simulink model "ModeAdjust"  (R2018b)
settings: Solver=FixedStepDiscrete  StartTime=0.0  StopTime=inf  FixedStep=0.01  RelTol=1e-3
undefined symbols (not defined in the file or in its folder): IfKeSMSbSeatMovBkRclnEnable_Val, IfKeSMSbSeatMovFrwdBkwdEnable_Val, IfKeSMSbSeatMovFtrstEnable_Val, IfKeSMSbSeatMovHdrstFrwdBkwdEnable_Val, IfKeSMSbSeatMovHdUpwdDnwdEnable_Val, IfKeSMSbSeatMovLgrstEnable_Val, IfKeSMSbSeatMovLtwdRtwdEnable_Val, IfVeSMSeStNumConfig, KeSMSbArmscreenMovEnable_Val, KeSMSbSeatMovLgrstExpdEnable_Val, KeSMSuFirstRwStBackPosDelta_Val, KeSMSuFirstRwStBackPosTolr_Val, KeSMSuFirstRwStCushFrntPosDelta_Val, KeSMSuFirstRwStCushFrntPosTolr_Val, KeSMSuFirstRwStCushRePosDelta_Val, KeSMSuFirstRwStCushRePosTolr_Val, KeSMSuFirstRwStFootrestPosDelta_Val, KeSMSuFirstRwStFootrestPosTolr_Val, KeSMSuFirstRwStFwdBkwdPosDelta_Val, KeSMSuFirstRwStFwdBkwdPosTolr_Val, KeSMSuMdMotFinshdTm_Val, KeSMSuMdRetryTm1_Val, KeSMSuModeReqDurgTm_Val, KeSMSuSecRwStArmTochPosDelta_Val, KeSMSuSecRwStArmTochPosTolr_Val, KeSMSuSecRwStBackPosDelta_Val, KeSMSuSecRwStBackPosTolr_Val, KeSMSuSecRwStFtrstUpwdDnwdPosDelta_Val, KeSMSuSecRwStFtrstUpwdDnwdPosTolr_Val, KeSMSuSecRwStFwdBkwdPosDelta_Val, KeSMSuSecRwStFwdBkwdPosTolr_Val, KeSMSuSecRwStHeadrestFwdBkwdPosDelta_Val, KeSMSuSecRwStHeadrestFwdBkwdPosTolr_Val, KeSMSuSecRwStHeadrestUpwdDwnwdPosDelta_Val, KeSMSuSecRwStHeadrestUpwdDwnwdPosTolr_Val, KeSMSuSecRwStLegrestInOutPosDelta_Val, KeSMSuSecRwStLegrestInOutPosTolr_Val, KeSMSuSecRwStLegrestUpwdDwnwdPosDelta_Val, KeSMSuSecRwStLegrestUpwdDwnwdPosTolr_Val, KeSMSuSecRwStLwdRwdPosDelta_Val, KeSMSuSecRwStLwdRwdPosTolr_Val, KeSMSuSecRwStVIPFtrstRefAngle_Val, KeSMSuThirdRwStFwdBkwdPosDelta_Val, KeSMSuThirdRwStFwdBkwdPosTolr_Val, KeSMSuThrdRwCushFoldPosDelta_Val, KeSMSuThrdRwCushFoldPosTolr_Val, KeSMSuThrdRwStBackPosDelta_Val, KeSMSuThrdRwStBackPosTolr_Val, KeSMSw4SLegrstCloseMdSecRwLtStFtrstUpwdDnwdPos_Val, KeSMSw4SLegrstCloseMdSecRwLtStFtrstUpwdDnwdPosMax_Val, KeSMSw4SLegrstCloseMdSecRwLtStFtrstUpwdDnwdPosMin_Val, KeSMSw4SLegrstCloseMdSecRwLtStLgrstOtwdInwdPos_Val, KeSMSw4SLegrstCloseMdSecRwLtStLgrstOtwdInwdPosMax_Val, KeSMSw4SLegrstCloseMdSecRwLtStLgrstOtwdInwdPosMin_Val, KeSMSw4SLegrstCloseMdSecRwLtStLgrstUpwdDnwdPos_Val, KeSMSw4SLegrstCloseMdSecRwLtStLgrstUpwdDnwdPosMax_Val, KeSMSw4SLegrstCloseMdSecRwLtStLgrstUpwdDnwdPosMin_Val, KeSMSw4SLegrstCloseMdSecRwRtStFtrstUpwdDnwdPos_Val, KeSMSw4SLegrstCloseMdSecRwRtStFtrstUpwdDnwdPosMax_Val, KeSMSw4SLegrstCloseMdSecRwRtStFtrstUpwdDnwdPosMin_Val ... (+1138)
libraries: Lib x401
(part 4 of 35)

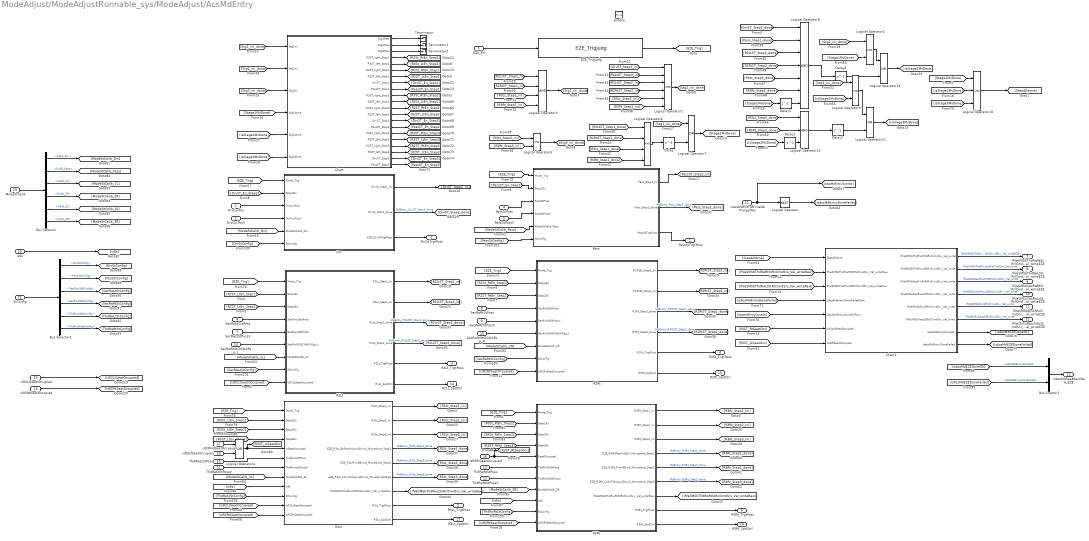
== system ModeAdjust/ModeAdjustRunnable_sys/ModeAdjust/AcsMdEntry ==
  EZE_En : Inport
  DrvCurPos : Inport  Port=2
  DrvCurPosV : Inport  Port=3
  PassStPoss : Inport  Port=4
  PassStPossV : Inport  Port=5
  SecRwLtStsPoss : Inport  Port=6
  SecRwLtStPossV : Inport  Port=7
  SecRwRtStPoss : Inport  Port=8
  SecRwRtStPossV : Inport  Port=9
  ThdRwLtStPoss : Inport  Port=10
  ThdRwLtStPossV : Inport  Port=11
  ThdRwRtStPoss : Inport  Port=12
  ThdRwRtStPossV : Inport  Port=13
  SecRwRtStChldLkRsp_L : Inport  Port=14
  SecRwRtStChldLkRsp_R : Inport  Port=15
  isR3RtSeatOccupied : Inport  Port=16
  isR3MidSeatOccupied : Inport  Port=17
  isR3LfSeatOccupied : Inport  Port=18
  ModeStCalib : Inport  Port=19
  is6s : Inport  Port=20
  StConfig : Inport  Port=21
  isAcsMdEntryArrivedAtTargetPos : Inport  Port=22
  isR2LtSeatOccupied : Inport  Port=23
  isR2RtSeatOccupied : Inport  Port=24
  Enable : EnablePort  StatesWhenEnabling=reset
  Bus Creator1 : BusCreator  Inputs=2
  Bus Selector : BusSelector  OutputSignals=Calib_Drv,Calib_Pass,Calib_2L,Calib_2R,Calib_3L,Calib_3R
  Bus Selector1 : BusSelector  OutputSignals=DrvStConfig,PassStConfig,SecRwLtStConfig,SecRwRtStConfig,ThdRwLtStConfig,ThdRwRtStConfig
  Chart : Stateflow chart  TreatAsAtomicUnit=on
  Chart1 : Stateflow chart  TreatAsAtomicUnit=on
  Delay{,1..4} (5 alike) : Delay  DelayLength=1
  Drv : Subsystem
  EZE_TrigJudg : Lib/EZE_TrigJudg  SystemSampleTime=-1
  Logical Operator : Logic  Operator=NOT  AllPortsSameDT=off  OutDataTypeStr=boolean
  Logical Operator1 : Logic  AllPortsSameDT=off  OutDataTypeStr=boolean
  Logical Operator{4,7,11,13} (4 alike) : Logic  Operator=OR  AllPortsSameDT=off  OutDataTypeStr=boolean
  Logical Operator12 : Logic  Inputs=3  AllPortsSameDT=off  OutDataTypeStr=boolean
  Logical Operator16 : Logic  Inputs=3  AllPortsSameDT=off  OutDataTypeStr=boolean
  Logical Operator2 : Logic  Inputs=6  AllPortsSameDT=off  OutDataTypeStr=boolean
  Logical Operator3 : Logic  Inputs=4  AllPortsSameDT=off  OutDataTypeStr=boolean
  Logical Operator5 : Logic  AllPortsSameDT=off  OutDataTypeStr=boolean
  Logical Operator6 : Logic  Inputs=4  AllPortsSameDT=off  OutDataTypeStr=boolean
  Logical Operator8 : Logic  Inputs=7  AllPortsSameDT=off  OutDataTypeStr=boolean
  Logical Operator9 : Logic  AllPortsSameDT=off  OutDataTypeStr=boolean
  Pass : Subsystem
  R2Lt : Subsystem
  R2Rt : Subsystem
  R3Lt : Subsystem
  R3Rt : Subsystem
  Terminator : Terminator
  Terminator1 : Terminator
  Terminator2 : Terminator
  DrvStTrgtPoss : Outport  VectorParamsAs1DForOutWhenUnconnected=on
  PassStTrgtPoss : Outport  Port=2  VectorParamsAs1DForOutWhenUnconnected=on
  R2Lt_TrgtPoss : Outport  Port=3  VectorParamsAs1DForOutWhenUnconnected=on
  R2Rt_TrgtPoss : Outport  Port=4  VectorParamsAs1DForOutWhenUnconnected=on
  R3Lt_TrgtPoss : Outport  Port=5  VectorParamsAs1DForOutWhenUnconnected=on
  R3Rt_TrgtPoss : Outport  Port=6  VectorParamsAs1DForOutWhenUnconnected=on
  IfVeSMSbThdRwRtStRclCmdSrv_Val_writeEZE : Outport  Port=7
  IfVeSMSbThdRwLtStRclCmdSrv_Val_writeEZE : Outport  Port=8
  IfVeSMSbSecRwRtStRclCmdSrv_Val_writeEZE : Outport  Port=9
  IfVeSMSuSecRwLtStRclCmdSrv_Val_writeEZE : Outport  Port=10
  IfVeSMSbDrvStRclCmdSrv_Val_writeEZE : Outport  Port=11
  IfVeSMSuPassStRclCmdSrv_Val_writeEZE : Outport  Port=12
  isAcsMdFeedBackNew_EZE : Outport  Port=13
  R2Lt_SpdCtrl : Outport  Port=14
  R2Rt_SpdCtrl : Outport  Port=15
  R3Rt_SpdCtrl : Outport  Port=16
  R3Lt_SpdCtrl : Outport  Port=17
  wires:
  EZE_En/1 -> EZE_TrigJudg/1
  EZE_TrigJudg/1 -> [EZE_Trig]
  [EZE_Trig] -> R3Rt/1(Mode_Trig)
  isR3LfSeatOccupied/1 -> Logical Operator4/2
  Logical Operator4/1 -> [R3ST_LtSeatOcc], R3Lt/5(isSeatOccupied)
  R3Rt/1(R3Rt_Step1_ini) -> [R3Rt_Step1_ini]
  R3Lt/1(R3Lt_Step1_ini) -> [R3Lt_Step1_ini]
  [Stg2_ini_done] -> Chart/2(Stg2ini)
  Chart/4(R3ST_right_Step1) -> [R3St_RtEn_Step1]
  [Stg1_ini_done] -> Chart/1(Stg1ini)
  [isStage3MvDone] -> Chart/6(Stg3done)
  [isStage2MvDone] -> Chart/5(Stg2done)
  [Stg3_ini_done] -> Chart/3(Stg3ini)
  [Stage1MvDone] -> Chart/4(Stg1done)
  Logical Operator5/1 -> [Stg3_ini_done]
  Logical Operator2/1 -> [Stg2_ini_done]
  Logical Operator3/1 -> [Stg1_ini_done]
  Chart/7(R2ST_left_Step1) -> [R2ST_LtEn_Step1]
  Chart/5(R3ST_left_Step1) -> [R3St_LtEn_Step1]
  Chart/6(R2ST_right_Step1) -> [R2St_RtEn_Step1]
  Chart/8(DrvST_Step1) -> [DrvST_En_Step1]
  Chart/9(PassST_Step1) -> [PassST_En_Step1]
  [PassST_En_Step2] -> Pass/2(Step1En)
  Logical Operator11/1 -> [isStage3MvDone]
  Logical Operator6/1 -> Delay/1
  Logical Operator7/1 -> [Stage1MvDone]
  [Stg1_ini_done] -> Logical Operator7/1
  Logical Operator13/1 -> [isStage2MvDone]
  Delay/1 -> Logical Operator7/2
  Logical Operator12/1 -> Delay2/1
  [R3Lt_Step3_done] -> Logical Operator12/1
  [R3Rt_Step3_done] -> Logical Operator12/2
  Logical Operator8/1 -> Delay4/1
  Drv/1(DrvSt_Step1_ini) -> [DrvST_Step2_ini]
  Pass/1(Pass_Step1_ini) -> [PassST_Step2_ini]
  R2Lt/1(R2Lt_Step1_Ini) -> [R2LtST_Step1_ini]
  R2Rt/1(R2RtSt_Step1_ini) -> [R2RtST_Step1_ini]
  R2Lt/2(R2Lt_Step2_Ini) -> [R2LtST_Step2_ini]
  R2Rt/2(R2RtSt_Step2_ini) -> [R2RtST_Step2_ini]
  R3Lt/2(R3Lt_Step2_ini) -> [R3Lt_Step2_ini]
  R3Rt/2(R3Rt_Step2_ini) -> [R3Rt_Step2_ini]
  R3Lt/3(R3Lt_Step3_ini) -> [R3Lt_Step3_ini]
  R3Rt/3(R3Rt_Step3_ini) -> [R3Rt_Step3_ini]
  [R3Lt_Step3_ini] -> Logical Operator5/1
  [R3Rt_Step3_ini] -> Logical Operator5/2
  Drv/2(DrvSt_Step1_done) -> [DrvST_Step2_done]  "MdEntry_DrvST_Step1_done"
  Pass/2(Pass_Step1_done) -> [Pass_Step2_done]  "MdEntry_Pass_Step1_done"
  R2Lt/3(R2Lt_Step1_done) -> [R2LtST_Step1_done]  "MdEntry_R2LtST_Step1_done"
  R2Lt/4(R2Lt_Step2_done) -> [R2LtST_Step2_done]  "MdEntry_R2LtST_Step2_done"
  R2Rt/3(R2Rt_Step1_done) -> [R2RtST_Step1_done]  "MdEntry_R2RtST_Step1_done"
  R2Rt/4(R2Rt_Step2_done) -> [R2RtST_Step2_done]  "MdEntry_R2RtST_Step2_done"
  R3Lt/4(EZE_R3Lt_BkReclnUpwdDnwd_Movedone_Step1) -> [R3Lt_Step1_done]  "MdEntry_R3Lt_Step1_done"
  R3Lt/5(EZE_R3LtFrwdBkwd_Movedone_Step2) -> [R3Lt_Step2_done]  "MdEntry_R3Lt_Step2_done"
  R3Lt/6(EZE_R3Lt_CshnFldUpwdDnwd_MovedoneStep3) -> [R3Lt_Step3_done]  "MdEntry_R3Lt_Step3_done"
  R3Rt/4(EZE_R3RtReclnUpDn_Movedone_Step1) -> [R3Rt_Step1_done]  "MdEntry_R3Rt_Step1_done"
  R3Rt/5(EZE_R3Rt_FrwdBkwd_Movedone_Step2) -> [R3Rt_Step2_done]  "MdEntry_R3Rt_Step2_done"
  R3Rt/6(EZE_R3Rt_CshnFldUpwdDnwd_Movedone_Step3) -> [R3Rt_Step3_done]  "MdEntry_R3Rt_Step3_done"
  [R2LtST_Step2_done] -> Logical Operator8/3
  [R3Lt_Step2_done] -> Logical Operator8/5
  [R3Rt_Step2_done] -> Logical Operator8/6
  R3Rt/7(IfVeSMSbThdRwRtStRclCmdSrv_Val_writeRaw) -> [IfVeSMSbThdRwRtStRclCmdSrv_Val_writeRaw]
  [IfVeSMSbThdRwRtStRclCmdSrv_Val_writeRaw] -> Chart1/2(IfVeSMSbThdRwRtStRclCmdSrv_Val_writeRaw)
  R3Lt/7(IfVeSMSbThdRwLtStRclCmdSrv_Val_writeRaw) -> [IfVeSMSbThdRwLtStRclCmdSrv_Val_writeRaw]
  [IfVeSMSbThdRwLtStRclCmdSrv_Val_writeRaw] -> Chart1/3(IfVeSMSbThdRwLtStRclCmdSrv_Val_writeRaw)
  [StepAlldone] -> Chart1/1(StepAlldone)
  Chart1/1(IfVeSMSbThdRwRtStRclCmdSrv_Val_write) -> IfVeSMSbThdRwRtStRclCmdSrv_Val_writeEZE/1  "IfVeSMSbThdRwRtStRclCmdSrv_Val_writeEZE"
  Chart1/2(IfVeSMSbThdRwLtStRclCmdSrv_Val_write) -> IfVeSMSbThdRwLtStRclCmdSrv_Val_writeEZE/1  "IfVeSMSbThdRwLtStRclCmdSrv_Val_write"
  Chart1/3(IfVeSMSbSecRwRtStRclCmdSrv_Val_write) -> IfVeSMSbSecRwRtStRclCmdSrv_Val_writeEZE/1  "IfVeSMSbSecRwRtStRclCmdSrv_Val_write"
  Chart1/4(IfVeSMSuSecRwLtStRclCmdSrv_Val_write) -> IfVeSMSuSecRwLtStRclCmdSrv_Val_writeEZE/1  "IfVeSMSuSecRwLtStRclCmdSrv_Val_write"
  Chart1/5(IfVeSMSbDrvStRclCmdSrv_Val_write) -> IfVeSMSbDrvStRclCmdSrv_Val_writeEZE/1  "IfVeSMSbDrvStRclCmdSrv_Val_write"
  Chart1/6(IfVeSMSuPassStRclCmdSrv_Val_write) -> IfVeSMSuPassStRclCmdSrv_Val_writeEZE/1  "IfVeSMSuPassStRclCmdSrv_Val_write"
  Chart/1(Stg1Req) -> Terminator/1
  Chart/2(Stg2Req) -> Terminator1/1
  Chart/3(Stg3Req) -> Terminator2/1
  isAcsMdEntryArrivedAtTargetPos/1 -> [isAcsMdEntryDoneOk], Logical Operator/1
  [isAcsMdEntryDoneOk] -> Chart1/5(isAcsMdEntryDoneOkRaw)
  [isAcsMdEntryDoneFailed] -> Chart1/4(isAcsMdEntryDoneFailedRaw)
  Chart1/7(isAcsMdEntryDoneOk) -> [isAcsMdEZEDoneOk]
  [EZE_Trig] -> Drv/1(Mode_Trig)
  [EZE_Trig] -> Pass/1(Mode_Trig)
  [EZE_Trig] -> R2Rt/1(Mode_Trig)
  [EZE_Trig] -> R2Lt/1(Mode_Trig)
  Drv/3(EZE_DrvStTrgtPoss) -> DrvStTrgtPoss/1
  Pass/3(PassStTrgtPoss) -> PassStTrgtPoss/1
  R2Lt/5(R2Lt_TrgtPoss) -> R2Lt_TrgtPoss/1
  R2Rt/5(R2Rt_TrgtPoss) -> R2Rt_TrgtPoss/1
  R3Lt/8(R3Lt_TrgtPoss) -> R3Lt_TrgtPoss/1
  [EZE_Trig] -> R3Lt/1(Mode_Trig)
  R3Rt/8(R3Rt_TrgtPoss) -> R3Rt_TrgtPoss/1
  DrvCurPos/1 -> Drv/3(DrvCurPos)
  DrvCurPosV/1 -> Drv/4(DrvCurPosV)
  PassStPoss/1 -> Pass/3(PassStPoss)
  PassStPossV/1 -> Pass/4(PassStPossV)
  SecRwLtStsPoss/1 -> R2Lt/4(SecRwLtStsPoss)
  SecRwLtStPossV/1 -> R2Lt/5(SecRwLtStPossV)
  ThdRwLtStPoss/1 -> R3Lt/6(ThdRwLtStPoss)
  ThdRwLtStPossV/1 -> R3Lt/7(ThdRwLtStPossV)
  ThdRwRtStPoss/1 -> R3Rt/6(ThdRwRtStPoss)
  ThdRwRtStPossV/1 -> R3Rt/7(ThdRwRtStPossV)
  SecRwRtStPoss/1 -> R2Rt/4(SecRwRtStPoss)
  SecRwRtStPossV/1 -> R2Rt/5(SecRwRtStPossV)
  isR3RtSeatOccupied/1 -> [R3ST_RtSeatOcc], R3Rt/5(SeatOccupied)
  SecRwRtStChldLkRsp_L/1 -> R2Lt/6(SecRwRtStChldLkRsp_L)
  SecRwRtStChldLkRsp_R/1 -> R2Rt/6(SecRwRtStChldLkRsp_L)
  isR3MidSeatOccupied/1 -> Logical Operator4/1
  [Stage1MvDone] -> Logical Operator16/1
  [isStage2MvDone] -> Logical Operator16/2
  [isStage3MvDone] -> Logical Operator16/3
  Chart/10(R3ST_right_Step2) -> [R3St_RtEn_Step2]
  Chart/11(R3ST_left_Step2) -> [R3St_LtEn_Step2]
  Chart/12(R2ST_right_Step2) -> [R2ST_RtEn_Step2]
  Chart/13(R2ST_left_Step2) -> [R2ST_LtEn_Step2]
  Chart/14(DrvST_Step2) -> [DrvST_En_Step2]
  Chart/15(PassST_Step2) -> [PassST_En_Step2]
  Chart/16(R3ST_right_Step3) -> [R3ST_RtEn_Step3]
  Chart/17(R3ST_left_Step3) -> [R3ST_LtEn_Step3]
  Chart/18(R2ST_right_Step3) -> [R2ST_RtEn_Step3]
  Chart/19(R2ST_left_Step3) -> [R2ST_LtEn_Step3]
  Chart/20(DrvST_Step3) -> [DrvST_En_Step3]
  Chart/21(PassST_Step3) -> [PassST_En_Step3]
  [DrvST_En_Step2] -> Drv/2(Step1En)
  [R2ST_LtEn_Step1] -> R2Lt/2(Step1En)
  [R2ST_LtEn_Step2] -> R2Lt/3(Step2En)
  [R2St_RtEn_Step1] -> R2Rt/2(Step1En)
  [R2ST_RtEn_Step2] -> R2Rt/3(Step2En)
  [R3ST_LtEn_Step3] -> R3Lt/4(Step3En)
  [R3St_LtEn_Step2] -> R3Lt/3(Step2En)
  [R3St_LtEn_Step1] -> R3Lt/2(Step1En)
  [R3ST_RtEn_Step3] -> R3Rt/4(Step3En)
  [R3St_RtEn_Step2] -> R3Rt/3(Step2En)
  [R3St_RtEn_Step1] -> R3Rt/2(Step1En)
  [isStage2MvDone] -> Delay1/1
  [Stage1MvDone] -> Delay3/1
  Chart1/8(isAcsMdEntryDoneFailed) -> [isAcsMdEZEDoneFailed]
  Logical Operator16/1 -> [StepAlldone]
  [R3ST_RtSeatOcc] -> Chart1/6(isRightSeatOccupied)
  [R3ST_LtSeatOcc] -> Chart1/7(isLeftSeatOccupied)
  ModeStCalib/1 -> Bus Selector/1
  Bus Selector/1 -> [ModeStCalib_Drv]  "<Calib_Drv>"
  Bus Selector/2 -> [ModeStCalib_Pass]  "<Calib_Pass>"
  Bus Selector/3 -> [ModeStCalib_2L]  "<Calib_2L>"
  Bus Selector/4 -> [ModeStCalib_2R]  "<Calib_2R>"
  Bus Selector/5 -> [ModeStCalib_3L]  "<Calib_3L>"
  Bus Selector/6 -> [ModeStCalib_3R]  "<Calib_3R>"
  [ModeStCalib_Drv] -> Drv/5(ModeStCalib_Drv)
  [ModeStCalib_Pass] -> Pass/5(ModeStCalib_Pass)
  [ModeStCalib_2L] -> R2Lt/7(ModeStCalib_2L)
  [ModeStCalib_2R] -> R2Rt/7(ModeStCalib_2R)
  [ModeStCalib_3L] -> R3Lt/8(ModeStCalib_3L)
  [ModeStCalib_3R] -> R3Rt/8(ModeStCalib_3R)
  is6s/1 -> [is6s]
  [is6s] -> R3Lt/9(is6s)
  [is6s] -> R3Rt/9(is6s)
  [isAcsMdEZEDoneOk] -> Bus Creator1/1  "isAcsMdEntryDoneOK"
  [isAcsMdEZEDoneFailed] -> Bus Creator1/2  "isAcsMdEntryDoneFailed"
  Bus Creator1/1 -> isAcsMdFeedBackNew_EZE/1
  StConfig/1 -> Bus Selector1/1
  Bus Selector1/1 -> [DrvStConfig]  "<DrvStConfig>"
  Bus Selector1/2 -> [PassStConfig]  "<PassStConfig>"
  Bus Selector1/3 -> [SecRwLtStConfig]  "<SecRwLtStConfig>"
  Bus Selector1/4 -> [SecRwRtStConfig]  "<SecRwRtStConfig>"
  Bus Selector1/5 -> [ThdRwLtStConfig]  "<ThdRwLtStConfig>"
  Bus Selector1/6 -> [ThdRwRtStConfig]  "<ThdRwRtStConfig>"
  [DrvStConfig] -> Drv/6(StConfig)
  [PassStConfig] -> Pass/6(StConfig)
  [SecRwLtStConfig] -> R2Lt/8(StConfig)
  [SecRwRtStConfig] -> R2Rt/8(StConfig)
  [ThdRwLtStConfig] -> R3Lt/10(StConfig)
  [ThdRwRtStConfig] -> R3Rt/10(StConfig)
  Logical Operator1/1 -> Logical Operator13/1
  [Stg2_ini_done] -> Logical Operator1/1
  [Stage1MvDone] -> Logical Operator1/2
  Delay3/1 -> Logical Operator8/7
  [Stg3_ini_done] -> Logical Operator9/1
  Logical Operator9/1 -> Logical Operator11/1
  [isStage2MvDone] -> Logical Operator9/2
  Delay1/1 -> Logical Operator12/3
  Delay2/1 -> Logical Operator11/2
  Delay4/1 -> Logical Operator13/2
  Logical Operator/1 -> [isAcsMdEntryDoneFailed]
  [R2RtST_Step2_done] -> Logical Operator8/4
  [R3Rt_Step2_ini] -> Logical Operator2/6
  [R3Lt_Step2_ini] -> Logical Operator2/5
  [R2RtST_Step2_ini] -> Logical Operator2/4
  [R2LtST_Step2_ini] -> Logical Operator2/3
  [DrvST_Step2_ini] -> Logical Operator2/1
  [DrvST_Step2_done] -> Logical Operator8/1
  [Pass_Step2_done] -> Logical Operator8/2
  [R3Rt_Step1_done] -> Logical Operator6/4
  [R2LtST_Step1_done] -> Logical Operator6/1
  [R2RtST_Step1_done] -> Logical Operator6/2
  [R3Lt_Step1_done] -> Logical Operator6/3
  [PassST_Step2_ini] -> Logical Operator2/2
  [R3Rt_Step1_ini] -> Logical Operator3/4
  [R3Lt_Step1_ini] -> Logical Operator3/3
  [R2RtST_Step1_ini] -> Logical Operator3/2
  [R2LtST_Step1_ini] -> Logical Operator3/1
  isR2LtSeatOccupied/1 -> [isR2LtSeatOccupied]
  isR2RtSeatOccupied/1 -> [isR2RtSeatOccupied]
  [isR2LtSeatOccupied] -> R2Lt/9(isR2LtSeatOccupied)
  [isR2RtSeatOccupied] -> R2Rt/9(isR2RtSeatOccupied)
  [isR2RtSeatOccupied] -> R3Rt/11(isR2RtSeatOccupied)
  [isR2LtSeatOccupied] -> R3Lt/11(isR2LtSeatOccupied)
  R2Lt/6(R2Lt_SpdCtrl) -> R2Lt_SpdCtrl/1
  R2Rt/6(R2Rt_SpdCtrl) -> R2Rt_SpdCtrl/1
  R3Rt/9(R3Rt_SpdCtrl) -> R3Rt_SpdCtrl/1
  R3Lt/9(R3Lt_SpdCtrl) -> R3Lt_SpdCtrl/1
  [isR2RtSeatOccupied] -> R3Lt/12(isR2RtSeatOccupied)

== system ModeAdjust/ModeAdjustRunnable_sys/ModeAdjust/AcsMdExt ==
  EZQ_En : Inport
  DrvCurPos : Inport  Port=2
  DrvCurPosV : Inport  Port=3
  PassStPoss : Inport  Port=4
  PassStPossV : Inport  Port=5
  SecRwLtStsPoss : Inport  Port=6
  SecRwLtStPossV : Inport  Port=7
  SecRwRtStPoss : Inport  Port=8
  SecRwRtStPossV : Inport  Port=9
  SecRwRtStChldLkRsp_L : Inport  Port=10
  SecRwRtStChldLkRsp_R : Inport  Port=11
  ModeStCalib : Inport  Port=12
  StConfig : Inport  Port=13
  isAcsMdExtArrivedAtTargetPosZone : Inport  Port=14
  isR2LtSeatOccupied : Inport  Port=15
  isR2RtSeatOccupied : Inport  Port=16
  Enable : EnablePort  StatesWhenEnabling=reset
  Bus Creator1 : BusCreator  Inputs=2
  Bus Selector : BusSelector  OutputSignals=Calib_Drv,Calib_Pass,Calib_2L,Calib_2R,Calib_3L,Calib_3R
  Bus Selector1 : BusSelector  OutputSignals=DrvStConfig,PassStConfig,SecRwLtStConfig,SecRwRtStConfig,ThdRwLtStConfig,ThdRwRtStConfig
  Chart : Stateflow chart  TreatAsAtomicUnit=on
  Chart1 : Stateflow chart  TreatAsAtomicUnit=on
  Delay : Delay  DelayLength=1
  Delay1 : Delay  DelayLength=1
  Delay2 : Delay  DelayLength=1
  Drv : Subsystem
  EZE_TrigJudg : Lib/EZE_TrigJudg  SystemSampleTime=-1
  Logical Operator : Logic  Operator=NOT  AllPortsSameDT=off  OutDataTypeStr=boolean
  Logical Operator13 : Logic  Operator=OR  AllPortsSameDT=off  OutDataTypeStr=boolean
  Logical Operator2 : Logic  Inputs=4  AllPortsSameDT=off  OutDataTypeStr=boolean
  Logical Operator{3..6} (4 alike) : Logic  AllPortsSameDT=off  OutDataTypeStr=boolean
  Logical Operator7 : Logic  Operator=OR  AllPortsSameDT=off  OutDataTypeStr=boolean
  Logical Operator8 : Logic  Inputs=5  AllPortsSameDT=off  OutDataTypeStr=boolean
  Pass : Subsystem
  R2Lt : Subsystem
  R2Rt : Subsystem
  Terminator : Terminator
  Terminator1 : Terminator
  DrvStTrgtPoss : Outport  VectorParamsAs1DForOutWhenUnconnected=on
  PassStTrgtPoss : Outport  Port=2  VectorParamsAs1DForOutWhenUnconnected=on
  R2Lt_TrgtPoss : Outport  Port=3  VectorParamsAs1DForOutWhenUnconnected=on
  R2Rt_TrgtPoss : Outport  Port=4  VectorParamsAs1DForOutWhenUnconnected=on
  IfVeSMSbSecRwRtStRclCmdSrv_Val_writeEZQ : Outport  Port=5
  IfVeSMSuSecRwLtStRclCmdSrv_Val_writeEZQ : Outport  Port=6
  IfVeSMSbDrvStRclCmdSrv_Val_writeEZQ : Outport  Port=7
  IfVeSMSuPassStRclCmdSrv_Val_writeEZQ : Outport  Port=8
  isAcsMdFeedBackNew_EZQ : Outport  Port=9
  R2Lt_SpdCtrl : Outport  Port=10
  R2Rt_SpdCtrl : Outport  Port=11
  wires:
  SecRwRtStChldLkRsp_R/1 -> R2Rt/6(SecRwRtStChldLkRsp_L)
  SecRwRtStChldLkRsp_L/1 -> R2Lt/6(SecRwRtStChldLkRsp_L)
  SecRwRtStPossV/1 -> R2Rt/5(SecRwRtStPossV)
  SecRwRtStPoss/1 -> R2Rt/4(SecRwRtStPoss)
  SecRwLtStPossV/1 -> R2Lt/5(SecRwLtStPossV)
  SecRwLtStsPoss/1 -> R2Lt/4(SecRwLtStsPoss)
  PassStPossV/1 -> Pass/4(PassStPossV)
  PassStPoss/1 -> Pass/3(PassStPoss)
  DrvCurPosV/1 -> Drv/4(DrvCurPosV)
  DrvCurPos/1 -> Drv/3(DrvCurPos)
  R2Rt/5(R2Rt_TrgtPoss) -> R2Rt_TrgtPoss/1
  R2Lt/5(R2Lt_TrgtPoss) -> R2Lt_TrgtPoss/1
  Pass/3(PassStTrgtPoss) -> PassStTrgtPoss/1
  Drv/3(EZE_DrvStTrgtPoss) -> DrvStTrgtPoss/1
  [EZE_Trig] -> R2Lt/1(Mode_Trig)
  [EZE_Trig] -> R2Rt/1(Mode_Trig)
  [EZE_Trig] -> Pass/1(Mode_Trig)
  [EZE_Trig] -> Drv/1(Mode_Trig)
  Chart1/5(isAcsMdEntryDoneOk) -> [isAcsMdQtDoneOk]
  Chart1/6(isAcsMdEntryDoneFailed) -> [isAcsMdQtDoneFailed]
  Logical Operator/1 -> [isAcsMdEntryDoneFailed]
  isAcsMdExtArrivedAtTargetPosZone/1 -> [isAcsMdEntryDoneOk], Logical Operator/1
  Chart/2(Stg2Req) -> Terminator1/1
  Chart/1(Stg1Req) -> Terminator/1
  [R2RtST_Step1_done] -> Logical Operator6/2
  [R2LtST_Step1_done] -> Logical Operator6/1
  R2Rt/4(R2Rt_Step2_done) -> [R2RtST_Step2_done]  "MdExt_R2RtST_Step2_done"
  R2Rt/3(R2Rt_Step1_done) -> [R2RtST_Step1_done]  "MdExt_R2RtST_Step1_done"
  R2Lt/4(R2Lt_Step2_done) -> [R2LtST_Step2_done]  "MdExt_R2LtST_Step2_done"
  R2Lt/3(R2Lt_Step1_done) -> [R2LtST_Step1_done]  "MdExt_R2LtST_Step1_done"
  Pass/2(Pass_Step1_done) -> [Pass_Step2_done]  "MdExt_Pass_Step1_done"
  Drv/2(DrvSt_Step1_done) -> [DrvST_Step2_done]  "MdExt_DrvST_Step1_done"
  R2Rt/2(R2RtSt_Step2_ini) -> [R2RtST_Step2_ini]
  R2Lt/2(R2Lt_Step2_Ini) -> [R2LtST_Step2_ini]
  R2Rt/1(R2RtSt_Step1_ini) -> [R2RtST_Step1_ini]
  R2Lt/1(R2Lt_Step1_Ini) -> [R2LtST_Step1_ini]
  Pass/1(Pass_Step1_ini) -> [PassST_Step2_ini]
  Drv/1(DrvSt_Step1_ini) -> [DrvST_Step2_ini]
  Logical Operator8/1 -> Delay1/1
  Delay/1 -> Logical Operator7/2
  Logical Operator13/1 -> [isStage2MvDone]
  [Stg1_ini_done] -> Logical Operator7/1
  Logical Operator7/1 -> [Stage1MvDone]
  Logical Operator6/1 -> Delay/1
  Chart/3(R2ST_right_Step1) -> [R2St_RtEn_Step1]
  Chart/4(R2ST_left_Step1) -> [R2ST_LtEn_Step1]
  Logical Operator3/1 -> [Stg1_ini_done]
  Logical Operator2/1 -> [Stg2_ini_done]
  [Stage1MvDone] -> Chart/3(Stg1done)
  [isStage2MvDone] -> Chart/4(Stg2done)
  [Stg1_ini_done] -> Chart/1(Stg1ini)
  [Stg2_ini_done] -> Chart/2(Stg2ini)
  EZE_TrigJudg/1 -> [EZE_Trig]
  EZQ_En/1 -> EZE_TrigJudg/1
  Chart/5(DrvST_Step1) -> [DrvST_En_Step1]
  Chart/6(PassST_Step1) -> [PassST_En_Step1]
  Chart/7(R2ST_right_Step2) -> [R2ST_RtEn_Step2]
  Chart/8(R2ST_left_Step2) -> [R2ST_LtEn_Step2]
  Chart/9(DrvST_Step2) -> [DrvST_En_Step2]
  Chart/10(PassST_Step2) -> [PassST_En_Step2]
  [DrvST_En_Step2] -> Drv/2(Step1En)
  [PassST_En_Step2] -> Pass/2(Step1En)
  [R2ST_LtEn_Step1] -> R2Lt/2(Step1En)
  [R2ST_LtEn_Step2] -> R2Lt/3(Step2En)
  [R2St_RtEn_Step1] -> R2Rt/2(Step1En)
  [R2ST_RtEn_Step2] -> R2Rt/3(Step2En)
  [isStage2MvDone] -> Logical Operator5/2
  [Stage1MvDone] -> Logical Operator5/1
  [Stage1MvDone] -> Delay2/1
  [isAcsMdEntryDoneOk] -> Chart1/7(isAcsMdEntryDoneOkRaw)
  [isAcsMdEntryDoneFailed] -> Chart1/6(isAcsMdEntryDoneFailedRaw)
  [IfVeSMSuSecRwLtStRclCmdSrv_Val_writeRaw] -> Chart1/3(IfVeSMSuSecRwLtStRclCmdSrv_Val_writeRaw)
  [IfVeSMSuPassStRclCmdSrv_Val_writeRaw] -> Chart1/5(IfVeSMSuPassStRclCmdSrv_Val_writeRaw)
  [IfVeSMSbDrvStRclCmdSrv_Val_writeRaw] -> Chart1/4(IfVeSMSbDrvStRclCmdSrv_Val_writeRaw)
  [IfVeSMSbSecRwRtStRclCmdSrv_Val_writeRaw] -> Chart1/2(IfVeSMSbSecRwRtStRclCmdSrv_Val_writeRaw)
  R2Rt/6(IfVeSMSbSecRwRtStRclCmdSrv_Val_writeRaw) -> [IfVeSMSbSecRwRtStRclCmdSrv_Val_writeRaw]
  R2Lt/6(IfVeSMSuSecRwLtStRclCmdSrv_Val_writeRaw) -> [IfVeSMSuSecRwLtStRclCmdSrv_Val_writeRaw]
  Drv/4(IfVeSMSbDrvStRclCmdSrv_Val_writeRaw) -> [IfVeSMSbDrvStRclCmdSrv_Val_writeRaw]
  Pass/4(IfVeSMSuPassStRclCmdSrv_Val_writeRaw) -> [IfVeSMSuPassStRclCmdSrv_Val_writeRaw]
  Chart1/1(IfVeSMSbSecRwRtStRclCmdSrv_Val_write) -> IfVeSMSbSecRwRtStRclCmdSrv_Val_writeEZQ/1  "IfVeSMSbSecRwRtStRclCmdSrv_Val_write"
  Chart1/4(IfVeSMSuPassStRclCmdSrv_Val_write) -> IfVeSMSuPassStRclCmdSrv_Val_writeEZQ/1  "IfVeSMSuPassStRclCmdSrv_Val_write"
  Chart1/3(IfVeSMSbDrvStRclCmdSrv_Val_write) -> IfVeSMSbDrvStRclCmdSrv_Val_writeEZQ/1  "IfVeSMSbDrvStRclCmdSrv_Val_write"
  Chart1/2(IfVeSMSuSecRwLtStRclCmdSrv_Val_write) -> IfVeSMSuSecRwLtStRclCmdSrv_Val_writeEZQ/1  "IfVeSMSuSecRwLtStRclCmdSrv_Val_write"
  Logical Operator5/1 -> [StageDone]
  [StageDone] -> Chart1/1(StepAlldone)
  Bus Selector/2 -> [ModeStCalib_Pass]  "<Calib_Pass>"
  Bus Selector/5 -> [ModeStCalib_3L]  "<Calib_3L>"
  Bus Selector/3 -> [ModeStCalib_2L]  "<Calib_2L>"
  Bus Selector/1 -> [ModeStCalib_Drv]  "<Calib_Drv>"
  Bus Selector/6 -> [ModeStCalib_3R]  "<Calib_3R>"
  Bus Selector/4 -> [ModeStCalib_2R]  "<Calib_2R>"
  ModeStCalib/1 -> Bus Selector/1
  [ModeStCalib_Drv] -> Drv/5(ModeStCalib_Drv)
  [ModeStCalib_Pass] -> Pass/5(ModeStCalib_Pass)
  [ModeStCalib_2L] -> R2Lt/7(ModeStCalib_2L)
  [ModeStCalib_2R] -> R2Rt/7(ModeStCalib_2R)
  [isAcsMdQtDoneOk] -> Bus Creator1/1  "isAcsMdExtDoneOK"
  [isAcsMdQtDoneFailed] -> Bus Creator1/2  "isAcsMdExtDoneFailed"
  Bus Creator1/1 -> isAcsMdFeedBackNew_EZQ/1
  Bus Selector1/6 -> [ThdRwRtStConfig]  "<ThdRwRtStConfig>"
  Bus Selector1/1 -> [DrvStConfig]  "<DrvStConfig>"
  Bus Selector1/3 -> [SecRwLtStConfig]  "<SecRwLtStConfig>"
  Bus Selector1/4 -> [SecRwRtStConfig]  "<SecRwRtStConfig>"
  StConfig/1 -> Bus Selector1/1
  Bus Selector1/2 -> [PassStConfig]  "<PassStConfig>"
  Bus Selector1/5 -> [ThdRwLtStConfig]  "<ThdRwLtStConfig>"
  [DrvStConfig] -> Drv/6(StConfig)
  [PassStConfig] -> Pass/6(StConfig)
  [SecRwLtStConfig] -> R2Lt/8(StConfig)
  [SecRwRtStConfig] -> R2Rt/8(StConfig)
  [Stg2_ini_done] -> Logical Operator4/1
  Logical Operator4/1 -> Logical Operator13/1
  [Stage1MvDone] -> Logical Operator4/2
  Delay1/1 -> Logical Operator13/2
  [R2RtST_Step2_ini] -> Logical Operator2/4
  [R2LtST_Step2_ini] -> Logical Operator2/3
  Delay2/1 -> Logical Operator8/5
  [R2RtST_Step2_done] -> Logical Operator8/4
  [R2LtST_Step2_done] -> Logical Operator8/3
  [R2LtST_Step1_ini] -> Logical Operator3/1
  [R2RtST_Step1_ini] -> Logical Operator3/2
  [PassST_Step2_ini] -> Logical Operator2/2
  [DrvST_Step2_ini] -> Logical Operator2/1
  [Pass_Step2_done] -> Logical Operator8/2
  [DrvST_Step2_done] -> Logical Operator8/1
  isR2LtSeatOccupied/1 -> [isR2LtSeatOccupied]
  isR2RtSeatOccupied/1 -> [isR2RtSeatOccupied]
  [isR2LtSeatOccupied] -> R2Lt/9(isR2LtSeatOccupied)
  [isR2RtSeatOccupied] -> R2Rt/9(isR2RtSeatOccupied)
  R2Lt/7(R2Lt_SpdCtrl) -> R2Lt_SpdCtrl/1
  R2Rt/7(R2Rt_SpdCtrl) -> R2Rt_SpdCtrl/1

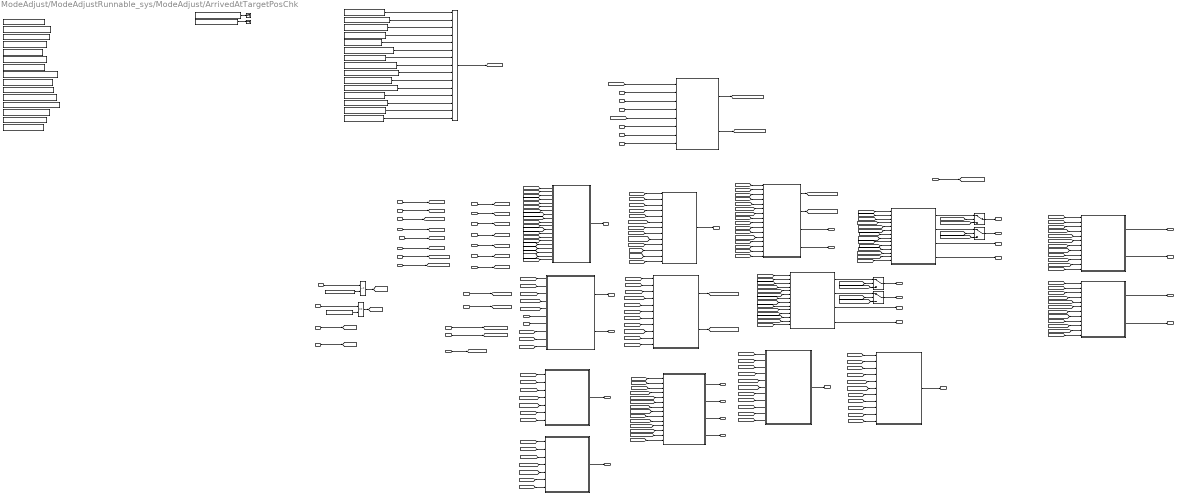
== system ModeAdjust/ModeAdjustRunnable_sys/ModeAdjust/ArrivedAtTargetPosChk ==
  note: %七座版
      | 包括左中占位
  note: %1锁，2未锁
  note: %1锁，2未锁
  DrvCurPos : Inport
  PassStPoss : Inport  Port=2
  SecRwLtStsPoss : Inport  Port=3
  SecRwRtStPoss : Inport  Port=4
  ThdRwLtStPoss : Inport  Port=5
  ThdRwRtStPoss : Inport  Port=6
  ModeStCalib : Inport  Port=7
  is6s : Inport  Port=8
  StConfig : Inport  Port=9
  SecRwLtStsPoss4s : Inport  Port=10
  SecRwRtStsPoss4s : Inport  Port=11
  StConfig4s : Inport  Port=12
  IfVeSMSbThdRwLtStFrwdCmdSrv_Val_read : Inport  Port=13
  IfVeSMSbThdRwRtStFrwdCmdSrv_Val_read : Inport  Port=14
  DrvCurPosV : Inport  Port=15
  PassStPossV : Inport  Port=16
  SecRwLtStsPossV : Inport  Port=17
  SecRwRtStPossV : Inport  Port=18
  ThdRwLtStPossV : Inport  Port=19
  ThdRwRtStPossV : Inport  Port=20
  SecRwLtStsPoss4sV : Inport  Port=21
  SecRwRtStsPoss4sV : Inport  Port=22
  SecRwLtStChldLkRsp_L : Inport  Port=23
  SecRwRtStChldLkRsp_R : Inport  Port=24
  R3LOccupied : Inport  Port=25
  R3ROccupied : Inport  Port=26
  is4s : Inport  Port=27
  VIP4sLEn : Inport  Port=28
  VIP4sREn : Inport  Port=29
  Rev4sLEn : Inport  Port=30
  Rev4sREn : Inport  Port=31
  Ly4sLEn : Inport  Port=32
  Ly4sREn : Inport  Port=33
  AcsMdEntry : Subsystem
  AcsMdExt : Subsystem
  Bus Creator : BusCreator  Inputs=15
  Check4sHeight : Subsystem
  FamlyL : Subsystem
  FamlyR : Subsystem
  INTML : Subsystem
  INTMR : Subsystem
  LgrstClose : Subsystem
  LgrstOpen : Subsystem
  Lug : Subsystem
  Ly : Subsystem
  PA_KeSMSuFirstRwStBackPosDelta_Val : Constant  Value=KeSMSuFirstRwStBackPosDelta_Val
  PA_KeSMSuFirstRwStBackPosTolr_Val : Constant  Value=KeSMSuFirstRwStBackPosTolr_Val
  PA_KeSMSuFirstRwStCushFrntPosTolr_Val : Constant  Value=KeSMSuFirstRwStCushFrntPosTolr_Val
  PA_KeSMSuFirstRwStCushRePosTolr_Val : Constant  Value=KeSMSuFirstRwStCushRePosTolr_Val
  PA_KeSMSuFirstRwStFootrestPosDelta_Val : Constant  Value=KeSMSuFirstRwStFootrestPosDelta_Val
  PA_KeSMSuFirstRwStFootrestPosTolr_Val : Constant  Value=KeSMSuFirstRwStFootrestPosTolr_Val
  PA_KeSMSuFirstRwStFwdBkwdPosDelta_Val : Constant  Value=KeSMSuFirstRwStFwdBkwdPosDelta_Val
  PA_KeSMSuFirstRwStFwdBkwdPosTolr_Val : Constant  Value=KeSMSuFirstRwStFwdBkwdPosTolr_Val
  PA_KeSMSuSecRwStArmTochPosDelta_Val : Constant  Value=KeSMSuSecRwStArmTochPosDelta_Val
  PA_KeSMSuSecRwStArmTochPosTolr_Val : Constant  Value=KeSMSuSecRwStArmTochPosTolr_Val
  PA_KeSMSuSecRwStBackPosDelta_Val : Constant  Value=KeSMSuSecRwStBackPosDelta_Val
  PA_KeSMSuSecRwStBackPosTolr_Val : Constant  Value=KeSMSuSecRwStBackPosTolr_Val
  PA_KeSMSuSecRwStFtrstUpwdDnwdPosDelta_Val : Constant  Value=KeSMSuSecRwStFtrstUpwdDnwdPosDelta_Val
  PA_KeSMSuSecRwStFtrstUpwdDnwdPosTolr_Val : Constant  Value=KeSMSuSecRwStFtrstUpwdDnwdPosTolr_Val
  PA_KeSMSuSecRwStFwdBkwdPosDelta_Val : Constant  Value=KeSMSuSecRwStFwdBkwdPosDelta_Val
  PA_KeSMSuSecRwStFwdBkwdPosTolr_Val : Constant  Value=KeSMSuSecRwStFwdBkwdPosTolr_Val
  PA_KeSMSuSecRwStHeadrestFwdBkwdPosDelta_Val : Constant  Value=KeSMSuSecRwStHeadrestFwdBkwdPosDelta_Val
  PA_KeSMSuSecRwStHeadrestFwdBkwdPosTolr_Val : Constant  Value=KeSMSuSecRwStHeadrestFwdBkwdPosTolr_Val
  PA_KeSMSuSecRwStHeadrestUpwdDwnwdPosDelta_Val : Constant  Value=KeSMSuSecRwStHeadrestUpwdDwnwdPosDelta_Val
  PA_KeSMSuSecRwStHeadrestUpwdDwnwdPosTolr_Val : Constant  Value=KeSMSuSecRwStHeadrestUpwdDwnwdPosTolr_Val
  PA_KeSMSuSecRwStLegrestInOutPosDelta_Val : Constant  Value=KeSMSuSecRwStLegrestInOutPosDelta_Val
  PA_KeSMSuSecRwStLegrestInOutPosTolr_Val : Constant  Value=KeSMSuSecRwStLegrestInOutPosTolr_Val
  PA_KeSMSuSecRwStLegrestUpwdDwnwdPosDelta_Val : Constant  Value=KeSMSuSecRwStLegrestUpwdDwnwdPosDelta_Val
  PA_KeSMSuSecRwStLegrestUpwdDwnwdPosTolr_Val : Constant  Value=KeSMSuSecRwStLegrestUpwdDwnwdPosTolr_Val
  PA_KeSMSuSecRwStLwdRwdPosDelta_Val : Constant  Value=KeSMSuSecRwStLwdRwdPosDelta_Val
  PA_KeSMSuSecRwStLwdRwdPosTolr_Val : Constant  Value=KeSMSuSecRwStLwdRwdPosTolr_Val
  PA_KeSMSuThirdRwStFwdBkwdPosDelta_Val : Constant  Value=KeSMSuThirdRwStFwdBkwdPosDelta_Val
  PA_KeSMSuThirdRwStFwdBkwdPosTolr_Val : Constant  Value=KeSMSuThirdRwStFwdBkwdPosTolr_Val
  PA_KeSMSuThrdRwCushFoldPosDelta_Val : Constant  Value=KeSMSuThrdRwCushFoldPosDelta_Val
  PA_KeSMSuThrdRwCushFoldPosTolr_Val : Constant  Value=KeSMSuThrdRwCushFoldPosTolr_Val
  PA_KeSMSuThrdRwStBackPosDelta_Val : Constant  Value=KeSMSuThrdRwStBackPosDelta_Val
  PA_KeSMSuThrdRwStBackPosTolr_Val : Constant  Value=KeSMSuThrdRwStBackPosTolr_Val
  PA_KeSMSwDltTrgtPos_Val1 : Constant  Value=SeatChldLkSt.ChldLkSt_Lock
  PA_KeSMSwDltTrgtPos_Val2 : Constant  Value=SeatChldLkSt.ChldLkSt_Unlock
  Recovery : Subsystem
  Recovery4s : Subsystem
  Relational Operator : RelationalOperator  Operator=~=  OutDataTypeStr=boolean  RndMeth=Simplest
  Relational Operator1 : RelationalOperator  Operator===  OutDataTypeStr=boolean  RndMeth=Simplest
  Switch{1..4} (4 alike) : Switch  Criteria=u2 > Threshold
  Terminator : Terminator
  Terminator1 : Terminator
  VIP : Subsystem
  Vip4s : Subsystem
  isAcsMdEntryArrivedAtTargetPos : Outport
  isAcsMdExtArrivedAtTargetPos : Outport  Port=2
  isLfVipArrivedAtTargetPos : Outport  Port=3
  isRtVipArrivedAtTargetPos : Outport  Port=4
  isLfLugArrivedAtTargetPos : Outport  Port=5
  isRtLugArrivedAtTargetPos : Outport  Port=6
  isLfRecoveryArrivedAtTargetPos : Outport  Port=7
  isRtRecoveryArrivedAtTargetPos : Outport  Port=8
  isINTMArrivedAtTargetPos : Outport  Port=9
  isLfFamlyArrivedAtTargetPos : Outport  Port=10
  isRtFamlyArrivedAtTargetPos : Outport  Port=11
  isLfLyArrivedAtTargetPos : Outport  Port=12
  isRtLyArrivedAtTargetPos : Outport  Port=13
  Drv_FtUpwdDnwdPosTrgt : Outport  Port=14
  PassSt_FtUpwdDnwdPosTrgt : Outport  Port=15
  isINTMRArrivedAtTargetPos : Outport  Port=16
  isLgrstOpenLArrivedAtTargetPos : Outport  Port=17
  isLgrstOpenRArrivedAtTargetPos : Outport  Port=18
  isLgrstCloseLArrivedAtTargetPos : Outport  Port=19
  isLgrstCloseRArrivedAtTargetPos : Outport  Port=20
  Calib_VIP4sLAdpt : Outport  Port=21
  Calib_VIP4sRAdpt : Outport  Port=22
  Calib_Recoery4sLAdpt : Outport  Port=23
  Calib_Recoery4sRAdpt : Outport  Port=24
  Calib_Ly4sLAdpt : Outport  Port=25
  Calib_Ly4sRAdpt : Outport  Port=26
  wires:
  DrvCurPos/1 -> [DrvCurPos]
  [DrvCurPos] -> AcsMdEntry/1(DrvCurPos)
  PassStPoss/1 -> [PassStPoss]
  SecRwLtStsPoss/1 -> [SecRwLtStsPoss]
  SecRwRtStPoss/1 -> [SecRwRtStPoss]
  ThdRwLtStPoss/1 -> [ThdRwLtStPoss]
  ThdRwRtStPoss/1 -> [ThdRwRtStPoss]
  [PassStPoss] -> AcsMdEntry/2(PassStPoss)
  [SecRwLtStsPoss] -> AcsMdEntry/3(SecRwLtStsPoss)
  [SecRwRtStPoss] -> AcsMdEntry/4(SecRwRtStPoss)
  [ThdRwLtStPoss] -> AcsMdEntry/5(ThdRwLtStPoss)
  [ThdRwRtStPoss] -> AcsMdEntry/6(ThdRwRtStPoss)
  AcsMdEntry/1(isAcsMdEntryArrivedAtTargetPos) -> isAcsMdEntryArrivedAtTargetPos/1
  [SecRwRtStPoss] -> AcsMdExt/4(SecRwRtStPoss)
  [SecRwLtStsPoss] -> AcsMdExt/3(SecRwLtStsPoss)
  [PassStPoss] -> AcsMdExt/2(PassStPoss)
  [DrvCurPos] -> AcsMdExt/1(DrvCurPos)
  AcsMdExt/1(isAcsMdExtArrivedAtTargetPos) -> isAcsMdExtArrivedAtTargetPos/1
  [SecRwLtStsPoss] -> VIP/1(SecRwLtStsPoss)
  [SecRwRtStPoss] -> VIP/2(SecRwRtStPoss)
  [ThdRwLtStPoss] -> VIP/3(ThdRwLtStPoss)
  [ThdRwRtStPoss] -> VIP/4(ThdRwRtStPoss)
  [ThdRwLtStPoss] -> Lug/1(ThdRwLtStPoss)
  [ThdRwRtStPoss] -> Lug/2(ThdRwRtStPoss)
  [SecRwLtStsPoss] -> Recovery/1(SecRwLtStsPoss)
  [SecRwRtStPoss] -> Recovery/2(SecRwRtStPoss)
  Lug/1(isLfLugArrivedAtTargetPos) -> isLfLugArrivedAtTargetPos/1
  Lug/2(isRtLugArrivedAtTargetPos) -> isRtLugArrivedAtTargetPos/1
  [ModeStCalib] -> AcsMdEntry/7(ModeStCalib)
  ModeStCalib/1 -> [ModeStCalib]
  [ModeStCalib] -> AcsMdExt/5(ModeStCalib)
  [ModeStCalib] -> Lug/3(ModeStCalib)
  [ModeStCalib] -> Recovery/3(ModeStCalib)
  [ModeStCalib] -> VIP/5(ModeStCalib)
  is6s/1 -> [is6s]
  [is6s] -> AcsMdEntry/8(is6s)
  [is6s] -> Lug/4(is6s)
  [is6s] -> VIP/6(is6s)
  StConfig/1 -> [StConfig]
  [StConfig] -> AcsMdEntry/9(StConfig)
  [StConfig] -> Lug/5(StConfig)
  [StConfig] -> Recovery/4(StConfig)
  [StConfig] -> AcsMdExt/6(StConfig)
  [StConfig] -> VIP/7(StConfig)
  [StConfig] -> FamlyL/5(StConfig)
  [ModeStCalib] -> FamlyL/4(ModeStCalib)
  FamlyL/1(isLfFamlyArrivedAtTargetPos) -> isLfFamlyArrivedAtTargetPos/1
  [ThdRwRtStPoss] -> FamlyL/3(ThdRwRtStPoss)
  [SecRwRtStPoss] -> FamlyL/2(SecRwRtStPoss)
  [SecRwLtStsPoss] -> FamlyL/1(SecRwLtStsPoss)
  [StConfig] -> INTML/4(StConfig)
  [ModeStCalib] -> INTML/3(ModeStCalib)
  INTML/1(isINTMArrivedAtTargetPos) -> isINTMArrivedAtTargetPos/1
  [SecRwRtStPoss] -> INTML/2(SecRwRtStPoss)
  [SecRwLtStsPoss] -> INTML/1(SecRwLtStsPoss)
  [SecRwLtStsPoss] -> Ly/1(SecRwLtStsPoss)
  [SecRwRtStPoss] -> Ly/2(SecRwRtStPoss)
  Ly/1(isLfRecoveryArrivedAtTargetPos) -> isLfLyArrivedAtTargetPos/1
  Ly/2(isRtRecoveryArrivedAtTargetPos) -> isRtLyArrivedAtTargetPos/1
  [ModeStCalib] -> Ly/3(ModeStCalib)
  [StConfig] -> Ly/4(StConfig)
  [SecRwLtStsPoss] -> FamlyR/1(SecRwLtStsPoss)
  [SecRwRtStPoss] -> FamlyR/2(SecRwRtStPoss)
  [ThdRwLtStPoss] -> FamlyR/3(ThdRwLtStPoss)
  FamlyR/1(isRtFamlyArrivedAtTargetPos) -> isRtFamlyArrivedAtTargetPos/1
  [ModeStCalib] -> FamlyR/4(ModeStCalib)
  [StConfig] -> FamlyR/5(StConfig)
  SecRwLtStsPoss4s/1 -> [SecRwLtStsPoss4s]
  SecRwRtStsPoss4s/1 -> [SecRwRtStsPoss4s]
  [SecRwLtStsPoss4s] -> Ly/5(SecRwLtStsPoss4s)
  [SecRwRtStsPoss4s] -> Ly/6(SecRwRtStsPoss4s)
  [StConfig4s] -> Ly/7(StConfig4s)
  StConfig4s/1 -> [StConfig4s]
  [StConfig4s] -> Vip4s/7(StConfig4s)
  [SecRwRtStsPoss4s] -> Vip4s/6(SecRwRtStsPoss4s)
  [SecRwLtStsPoss4s] -> Vip4s/5(SecRwLtStsPoss4s)
  [StConfig] -> Vip4s/4(StConfig)
  [ModeStCalib] -> Vip4s/3(ModeStCalib)
  [SecRwRtStPoss] -> Vip4s/2(SecRwRtStPoss)
  [SecRwLtStsPoss] -> Vip4s/1(SecRwLtStsPoss)
  Vip4s/1(isLfRecoveryArrivedAtTargetPos) -> Switch1/1
  [isLfVipArrivedAtTargetPos] -> Switch1/3
  is4s/1 -> [is4s]
  Switch1/1 -> isLfVipArrivedAtTargetPos/1
  [is4s] -> Switch1/2
  Switch2/1 -> isRtVipArrivedAtTargetPos/1
  [is4s] -> Switch2/2
  Vip4s/2(isRtRecoveryArrivedAtTargetPos) -> Switch2/1
  VIP/1(isLfVipArrivedAtTargetPos) -> [isLfVipArrivedAtTargetPos]
  VIP/2(isRtVipArrivedAtTargetPos) -> [isRtVipArrivedAtTargetPos]
  [isRtVipArrivedAtTargetPos] -> Switch2/3
  [StConfig4s] -> Recovery4s/7(StConfig4s)
  [SecRwRtStsPoss4s] -> Recovery4s/6(SecRwRtStsPoss4s)
  [SecRwLtStsPoss4s] -> Recovery4s/5(SecRwLtStsPoss4s)
  [StConfig] -> Recovery4s/4(StConfig)
  [ModeStCalib] -> Recovery4s/3(ModeStCalib)
  [SecRwRtStPoss] -> Recovery4s/2(SecRwRtStPoss)
  [SecRwLtStsPoss] -> Recovery4s/1(SecRwLtStsPoss)
  [isLfRecoveryArrivedAtTargetPos] -> Switch3/3
  Recovery4s/1(isLfRecoveryArrivedAtTargetPos) -> Switch3/1
  [is4s] -> Switch3/2
  Switch3/1 -> isLfRecoveryArrivedAtTargetPos/1
  [is4s] -> Switch4/2
  Recovery4s/2(isRtRecoveryArrivedAtTargetPos) -> Switch4/1
  [isRtRecoveryArrivedAtTargetPos] -> Switch4/3
  Switch4/1 -> isRtRecoveryArrivedAtTargetPos/1
  Recovery/1(isLfRecoveryArrivedAtTargetPos) -> [isLfRecoveryArrivedAtTargetPos]
  Recovery/2(isRtRecoveryArrivedAtTargetPos) -> [isRtRecoveryArrivedAtTargetPos]
  [DrvCurPos] -> Recovery/5(DrvCurPos)
  [PassStPoss] -> Recovery/6(PassStPoss)
  [PassStPoss] -> VIP/9(PassStPoss)
  [DrvCurPos] -> VIP/8(DrvCurPos)
  IfVeSMSbThdRwLtStFrwdCmdSrv_Val_read/1 -> Lug/6(IfVeSMSbThdRwLtStFrwdCmdSrv_Val_read)
  IfVeSMSbThdRwRtStFrwdCmdSrv_Val_read/1 -> Lug/7(IfVeSMSbThdRwRtStFrwdCmdSrv_Val_read)
  DrvCurPosV/1 -> [DrvCurPosV]
  PassStPossV/1 -> [PassStPossV]
  SecRwLtStsPossV/1 -> [SecRwLtStsPossV]
  SecRwRtStPossV/1 -> [SecRwRtStPossV]
  ThdRwLtStPossV/1 -> [ThdRwLtStPossV]
  ThdRwRtStPossV/1 -> [ThdRwRtStPossV]
  SecRwLtStsPoss4sV/1 -> [SecRwLtStsPoss4sV]
  SecRwRtStsPoss4sV/1 -> [SecRwRtStsPoss4sV]
  [ThdRwLtStPossV] -> AcsMdEntry/14(ThdRwLtStPossV)
  [ThdRwRtStPossV] -> AcsMdEntry/15(ThdRwRtStPossV)
  [SecRwLtStsPossV] -> AcsMdEntry/12(SecRwLtStsPossV)
  [SecRwRtStPossV] -> AcsMdEntry/13(SecRwRtStPossV)
  [PassStPossV] -> AcsMdEntry/11(PassStPossV)
  [DrvCurPosV] -> AcsMdEntry/10(DrvCurPosV)
  [ChildLockerL] -> AcsMdEntry/16(ChildLockerL)
  Relational Operator/1 -> [ChildLockerL]
  PA_KeSMSwDltTrgtPos_Val2/1 -> Relational Operator/2
  SecRwLtStChldLkRsp_L/1 -> Relational Operator/1
  SecRwRtStChldLkRsp_R/1 -> Relational Operator1/1
  Relational Operator1/1 -> [ChildLockerR]
  PA_KeSMSwDltTrgtPos_Val1/1 -> Relational Operator1/2
  [ChildLockerR] -> AcsMdEntry/17(ChildLockerR)
  R3LOccupied/1 -> [R3LOccupied]
  R3ROccupied/1 -> [R3ROccupied]
  [R3LOccupied] -> AcsMdEntry/18(R3LOccupied)
  [R3ROccupied] -> AcsMdEntry/19(R3ROccupied)
  [SecRwLtStsPossV] -> AcsMdExt/9(SecRwLtStsPossV)
  [PassStPossV] -> AcsMdExt/8(PassStPossV)
  [SecRwRtStPossV] -> AcsMdExt/10(SecRwRtStPossV)
  [DrvCurPosV] -> AcsMdExt/7(DrvCurPosV)
  [ChildLockerL] -> AcsMdExt/11(ChildLockerL)
  [ChildLockerR] -> AcsMdExt/12(ChildLockerR)
  [ThdRwRtStPossV] -> Lug/9(ThdRwRtStPossV)
  [ThdRwLtStPossV] -> Lug/8(ThdRwLtStPossV)
  [DrvCurPosV] -> Recovery/7(DrvCurPosV)
  [PassStPossV] -> Recovery/8(PassStPossV)
  [SecRwLtStsPossV] -> Recovery/9(SecRwLtStsPossV)
  [SecRwRtStPossV] -> Recovery/10(SecRwRtStPossV)
  [SecRwRtStPossV] -> INTML/6(SecRwRtStPossV)
  [SecRwLtStsPossV] -> INTML/5(SecRwLtStsPossV)
  [SecRwLtStsPossV] -> Ly/8(SecRwLtStsPossV)
  [SecRwRtStPossV] -> Ly/9(SecRwRtStPossV)
  [SecRwLtStsPoss4sV] -> Ly/10(SecRwLtStsPoss4sV)
  [SecRwRtStsPoss4sV] -> Ly/11(SecRwRtStsPoss4sV)
  [SecRwRtStPossV] -> Recovery4s/9(SecRwRtStPossV)
  [SecRwRtStsPoss4sV] -> Recovery4s/11(SecRwRtStsPoss4sV)
  [SecRwLtStsPossV] -> Recovery4s/8(SecRwLtStsPossV)
  [SecRwLtStsPoss4sV] -> Recovery4s/10(SecRwLtStsPoss4sV)
  [SecRwRtStPossV] -> Vip4s/9(SecRwRtStPossV)
  [SecRwLtStsPoss4sV] -> Vip4s/10(SecRwLtStsPoss4sV)
  [SecRwRtStsPoss4sV] -> Vip4s/11(SecRwRtStsPoss4sV)
  [SecRwLtStsPossV] -> Vip4s/8(SecRwLtStsPossV)
  [DrvCurPosV] -> VIP/10(DrvCurPosV)
  [SecRwRtStPossV] -> VIP/13(SecRwRtStPossV)
  [PassStPossV] -> VIP/11(PassStPossV)
  [ThdRwRtStPossV] -> VIP/15(ThdRwRtStPossV)
  [ThdRwLtStPossV] -> VIP/14(ThdRwLtStPossV)
  [SecRwLtStsPossV] -> VIP/12(SecRwLtStsPossV)
  [SecRwLtStsPossV] -> FamlyL/6(SecRwLtStsPossV)
  [SecRwRtStPossV] -> FamlyL/7(SecRwRtStPossV)
  [ThdRwRtStPossV] -> FamlyL/8(ThdRwRtStPossV)
  [SecRwLtStsPossV] -> FamlyR/6(SecRwLtStsPossV)
  [SecRwRtStPossV] -> FamlyR/7(SecRwRtStPossV)
  [ThdRwLtStPossV] -> FamlyR/8(ThdRwLtStPossV)
  VIP/3(Drv_FtUpwdDnwdPosTrgt) -> Drv_FtUpwdDnwdPosTrgt/1
  VIP/4(PassSt_FtUpwdDnwdPosTrgt) -> PassSt_FtUpwdDnwdPosTrgt/1
  [SecRwLtStsPossV] -> INTMR/5(SecRwLtStsPossV)
  [SecRwRtStPossV] -> INTMR/6(SecRwRtStPossV)
  [SecRwLtStsPoss] -> INTMR/1(SecRwLtStsPoss)
  [SecRwRtStPoss] -> INTMR/2(SecRwRtStPoss)
  INTMR/1(isINTMArrivedAtTargetPos) -> isINTMRArrivedAtTargetPos/1
  [ModeStCalib] -> INTMR/3(ModeStCalib)
  [StConfig] -> INTMR/4(StConfig)
  [ThdRwLtStPossV] -> FamlyL/10(ThdRwLtStPossV)
  [ThdRwRtStPossV] -> FamlyR/10(ThdRwRtStPossV)
  [ThdRwLtStPoss] -> FamlyL/9(ThdRwLtStPoss)
  [ThdRwRtStPoss] -> FamlyR/9(ThdRwRtStPoss)
  LgrstOpen/2(isRtRecoveryArrivedAtTargetPos) -> isLgrstOpenRArrivedAtTargetPos/1
  [SecRwLtStsPoss] -> LgrstOpen/1(SecRwLtStsPoss)
  [SecRwLtStsPossV] -> LgrstOpen/8(SecRwLtStsPossV)
  [SecRwRtStPossV] -> LgrstOpen/9(SecRwRtStPossV)
  [SecRwRtStsPoss4sV] -> LgrstOpen/11(SecRwRtStsPoss4sV)
  LgrstOpen/1(isLfRecoveryArrivedAtTargetPos) -> isLgrstOpenLArrivedAtTargetPos/1
  [SecRwLtStsPoss4sV] -> LgrstOpen/10(SecRwLtStsPoss4sV)
  [ModeStCalib] -> LgrstOpen/3(ModeStCalib)
  [SecRwRtStsPoss4s] -> LgrstOpen/6(SecRwRtStsPoss4s)
  [StConfig4s] -> LgrstOpen/7(StConfig4s)
  [SecRwRtStPoss] -> LgrstOpen/2(SecRwRtStPoss)
  [StConfig] -> LgrstOpen/4(StConfig)
  [SecRwLtStsPoss4s] -> LgrstOpen/5(SecRwLtStsPoss4s)
  [SecRwLtStsPoss4sV] -> LgrstClose/10(SecRwLtStsPoss4sV)
  [SecRwLtStsPossV] -> LgrstClose/8(SecRwLtStsPossV)
  [SecRwRtStsPoss4sV] -> LgrstClose/11(SecRwRtStsPoss4sV)
  [SecRwRtStPossV] -> LgrstClose/9(SecRwRtStPossV)
  LgrstClose/2(isRtRecoveryArrivedAtTargetPos) -> isLgrstCloseRArrivedAtTargetPos/1
  LgrstClose/1(isLfRecoveryArrivedAtTargetPos) -> isLgrstCloseLArrivedAtTargetPos/1
  [SecRwLtStsPoss] -> LgrstClose/1(SecRwLtStsPoss)
  [SecRwRtStPoss] -> LgrstClose/2(SecRwRtStPoss)
  [ModeStCalib] -> LgrstClose/3(ModeStCalib)
  [StConfig] -> LgrstClose/4(StConfig)
  [SecRwLtStsPoss4s] -> LgrstClose/5(SecRwLtStsPoss4s)
  [SecRwRtStsPoss4s] -> LgrstClose/6(SecRwRtStsPoss4s)
  [StConfig4s] -> LgrstClose/7(StConfig4s)
  Vip4s/4(Calib_VIP4sRAdpt) -> Calib_VIP4sRAdpt/1
  Vip4s/3(Calib_VIP4sLAdpt) -> Calib_VIP4sLAdpt/1
  [SecRwLtStsPoss] -> Check4sHeight/1(SecRwLtStsPoss)
  Rev4sLEn/1 -> Check4sHeight/2(Rev4sLEn)
  Ly4sLEn/1 -> Check4sHeight/3(Ly4sLEn)
  VIP4sLEn/1 -> Check4sHeight/4(VIP4sLEn)
  [SecRwRtStPoss] -> Check4sHeight/5(SecRwRtStPoss)
  Rev4sREn/1 -> Check4sHeight/6(Rev4sREn)
  Ly4sREn/1 -> Check4sHeight/7(Ly4sREn)
  VIP4sREn/1 -> Check4sHeight/8(VIP4sREn)
  Check4sHeight/1(Lt4sHightIndex) -> [Lt4sHightIndex]
  Check4sHeight/2(Rt4sHightIndex) -> [Rt4sHightIndex]
  [Lt4sHightIndex] -> Vip4s/12(Lt4sHightIndex)
  [Rt4sHightIndex] -> Vip4s/13(Rt4sHightIndex)
  [Lt4sHightIndex] -> Recovery4s/12(Lt4sHightIndex)
  [Rt4sHightIndex] -> Recovery4s/13(Rt4sHightIndex)
  [Lt4sHightIndex] -> Ly/12(Lt4sHightIndex)
  [Rt4sHightIndex] -> Ly/13(Rt4sHightIndex)
  Recovery4s/4(Calib_Recoery4sRAdpt) -> Calib_Recoery4sRAdpt/1
  Recovery4s/3(Calib_Recoery4sLAdpt) -> Calib_Recoery4sLAdpt/1
  Ly/3(Calib_Ly4sLAdpt) -> Calib_Ly4sLAdpt/1
  Ly/4(Calib_Ly4sRAdpt) -> Calib_Ly4sRAdpt/1
  PA_KeSMSuSecRwStLwdRwdPosTolr_Val/1 -> Bus Creator/12  "KeSMSuSecRwStHeadrestUpwdDwnwdPosDelta_Val"
  PA_KeSMSuSecRwStLegrestUpwdDwnwdPosTolr_Val/1 -> Bus Creator/11  "KeSMSuSecRwStHeadrestFwdBkwdPosDelta_Val"
  PA_KeSMSuSecRwStHeadrestFwdBkwdPosTolr_Val/1 -> Bus Creator/8  "KeSMSuSecRwStLegrestUpwdDwnwdPosDelta_Val"
  PA_KeSMSuSecRwStLegrestInOutPosTolr_Val/1 -> Bus Creator/10  "KeSMSuSecRwStFtrstUpwdDnwdPosDelta_Val"
  PA_KeSMSuSecRwStHeadrestUpwdDwnwdPosTolr_Val/1 -> Bus Creator/9  "KeSMSuSecRwStLegrestInOutPosDelta_Val"
  PA_KeSMSuThirdRwStFwdBkwdPosTolr_Val/1 -> Bus Creator/13  "KeSMSuThirdRwStFwdBkwdPosDelta_Val"
  PA_KeSMSuThrdRwCushFoldPosTolr_Val/1 -> Bus Creator/14  "KeSMSuThrdRwCushFoldPosDelta_Val"
  PA_KeSMSuFirstRwStFootrestPosTolr_Val/1 -> Bus Creator/2  "KeSMSuFirstRwStFootrestPosDelta_Val"
  PA_KeSMSuSecRwStFtrstUpwdDnwdPosTolr_Val/1 -> Bus Creator/6  "KeSMSuSecRwStFwdBkwdPosDelta_Val"
  PA_KeSMSuFirstRwStFwdBkwdPosTolr_Val/1 -> Bus Creator/3  "KeSMSuFirstRwStFwdBkwdPosDelta_Val"
  PA_KeSMSuThrdRwStBackPosTolr_Val/1 -> Bus Creator/15  "KeSMSuThrdRwStBackPosDelta_Val"
  PA_KeSMSuSecRwStArmTochPosTolr_Val/1 -> Bus Creator/4  "KeSMSuSecRwStArmTochPosDelta_Val"
  PA_KeSMSuSecRwStFwdBkwdPosTolr_Val/1 -> Bus Creator/7  "KeSMSuSecRwStLwdRwdPosDelta_Val"
  PA_KeSMSuSecRwStBackPosTolr_Val/1 -> Bus Creator/5  "KeSMSuSecRwStBackPosDelta_Val"
  PA_KeSMSuFirstRwStBackPosTolr_Val/1 -> Bus Creator/1  "KeSMSuFirstRwStBackPosDelta_Val"
  Bus Creator/1 -> [PosDeltaCalib]
  [PosDeltaCalib] -> AcsMdEntry/20(PosDeltaCalib)
  [PosDeltaCalib] -> AcsMdExt/13(PosDeltaCalib)
  [PosDeltaCalib] -> VIP/16(PosDeltaCalib)
  [PosDeltaCalib] -> Vip4s/14(PosDeltaCalib)
  [PosDeltaCalib] -> LgrstOpen/12(PosDeltaCalib)
  [PosDeltaCalib] -> LgrstClose/12(PosDeltaCalib)
  [PosDeltaCalib] -> FamlyR/11(PosDeltaCalib)
  [PosDeltaCalib] -> FamlyL/11(PosDeltaCalib)
  [PosDeltaCalib] -> Recovery4s/14(PosDeltaCalib)
  [PosDeltaCalib] -> Recovery/11(PosDeltaCalib)
  [PosDeltaCalib] -> Lug/10(PosDeltaCalib)
  [PosDeltaCalib] -> INTML/7(PosDeltaCalib)
  [PosDeltaCalib] -> INTMR/7(PosDeltaCalib)
  [PosDeltaCalib] -> Ly/14(PosDeltaCalib)
  PA_KeSMSuFirstRwStCushFrntPosTolr_Val/1 -> Terminator/1
  PA_KeSMSuFirstRwStCushRePosTolr_Val/1 -> Terminator1/1
